simulink model "HDVSim_BEV_Truck"  (R2019b)
settings: Solver=ode3  StartTime=0.0  StopTime=inf  FixedStep=sample_time  MaxStep=0.1  RelTol=1e-3  EnableMultiTasking=on
model workspace (MAT data in the model file):
  Bat : object (value not decoded)
  Electric_Truck = 1
  FuelCell : P_nom (value not decoded)
  Fueltype = 7
  Hybrid_Truck = 1
  IZ12 = 3600
  M_el = 1000
  SOC_T_EM_completely_available = 0.5
  SOC_addition = 0.4
  SOC_el = 0.8
  SOC_target = 0.85
  Sailing_without_drag_torque = 0
  TCO : object (value not decoded)
  TCO_Trailer = 1
  T_distance_LPS_down = 250
  T_distance_LPS_up = 250
  VSim : object (value not decoded)
  Vehicle = 'empty'
  WPT : object (value not decoded)
  acquisitionCosts : acquisitionCosts (value not decoded)
  addition_for_critical_slope = 0.01
  ambient : object (value not decoded)
  auxiliary_consumers : object (value not decoded)
  critical_altitude_difference = 50
  cycle : object (value not decoded)
  dcycle = 22
  distance_1_PPC = 175
  distance_2_PPC = 200
  distance_PPC_altitude_difference = 10000
  driver : object (value not decoded)
  em : object (value not decoded)
  engine : object (value not decoded)
  final_drive : object (value not decoded)
  ifElectric = 1
  ifOptimized = 0
  look_ahead_PPC = 250
  max_distance = 100000
  name = 'HDVSim_BEV_Truck'
  preditiveCruiseControl = 0
  sample_time = 0.1
  tank : object (value not decoded)
  tires : object (value not decoded)
  transmission : object (value not decoded)
  v_PPC_delta = 2.77777777778
  v_max_electrical_drive_only = 13.8888888889
  vehicle : object (value not decoded)
  vehicleProperties : vehicleProperties (value not decoded)
  weights : weights (value not decoded)
  x = 1
values from neighbouring files (symbols this model uses):
  transmission = Transmission_gearing(15.86, 7, 0, 0, final_drive.ratio)    [Parameterizing.m]
symbols that are objects in the model workspace (value not decoded): ambient, auxiliary_consumers, Bat, cycle, driver, em, final_drive, tires, vehicle
undefined symbols (not defined in the file or in its folder): Ion, Lithium, prospective_cruise_control, Vorausschauender_Tempomat
libraries: simulink x21, powerlib x2, electricdrivelib x1
(part 3 of 3)

== system HDVSim_BEV_Truck/Active cruise control_old/Estimate acceleration/Fahrwiderstaende ohne Beschleunigung/drag - Luftwiderstand ==
  v [m/s] : Inport
  A : Constant  Value=vehicle.frontal_area
  Product2 : Product  Inputs=4  RndMeth=Zero
  cW : Constant  Value=vehicle.air_drag_coeff
  gain2 : Gain  Gain=0.5
  rho : Constant  Value=ambient.air_density
  v² : Math  Operator=square  SaturateOnIntegerOverflow=on
  F_Luft [N] : Outport  VectorParamsAs1DForOutWhenUnconnected=off
  wires:
  v²/1 -> Product2/1
  gain2/1 -> F_Luft [N]/1
  v [m/s]/1 -> v²/1
  rho/1 -> Product2/2
  A/1 -> Product2/3
  cW/1 -> Product2/4
  Product2/1 -> gain2/1

== system HDVSim_BEV_Truck/Active cruise control_old/Estimate acceleration/Fahrwiderstaende ohne Beschleunigung/grade resistance - Steigungswiderstand ==
  alpha [rad] : Inport
  Add : Sum
  Constant1 : Constant  Value=vehicle.payload
  Constant2 : Constant  Value=vehicle.mass
  Product7 : Product  RndMeth=Zero
  Trigonometric Function : Trigonometry
  g : Gain  Gain=ambient.gravity
  F_Steig [N] : Outport  VectorParamsAs1DForOutWhenUnconnected=off
  wires:
  alpha [rad]/1 -> Trigonometric Function/1
  Trigonometric Function/1 -> Product7/2
  Product7/1 -> F_Steig [N]/1
  g/1 -> Product7/1
  Constant2/1 -> Add/1
  Constant1/1 -> Add/2
  Add/1 -> g/1

== system HDVSim_BEV_Truck/Active cruise control_old/Estimate acceleration/Fahrwiderstaende ohne Beschleunigung/rolling resistance - Rollwiderstand ==
  alpha [rad] : Inport
  Add1 : Sum
  Constant1 : Constant  Value=vehicle.payload
  Constant5 : Constant  Value=tires.roll_drag_coeff.total
  Constant8 : Constant  Value=vehicle.mass
  Product7 : Product  Inputs=3  RndMeth=Zero
  Trigonometric Function : Trigonometry  Operator=cos
  g : Gain  Gain=ambient.gravity
  F_Roll [N] : Outport  VectorParamsAs1DForOutWhenUnconnected=off
  wires:
  alpha [rad]/1 -> Trigonometric Function/1
  Product7/1 -> F_Roll [N]/1
  Constant5/1 -> Product7/3
  Trigonometric Function/1 -> Product7/1
  g/1 -> Product7/2
  Constant8/1 -> Add1/1
  Constant1/1 -> Add1/2
  Add1/1 -> g/1

== system HDVSim_BEV_Truck/Transmission/Determine when shifting occurs/Gear change recommendation/recommend_down_calcbsfc1 ==
  n_ICE [rpm] : Inport
  shift_parameter.n_2 : Inport  Port=2
  delta_v : Inport  Port=3
  Compare To Constant : simulink/Logic and Bit Operations/Compare To Constant  relop=>=  const=8  OutDataTypeStr=boolean
  Compare To Constant1 : simulink/Logic and Bit Operations/Compare To Constant  relop=>=  const=5  OutDataTypeStr=boolean
  Compare To Zero3 : simulink/Logic and Bit Operations/Compare To Zero  relop=<=  OutDataTypeStr=boolean
  Constant : Constant  Value=em.n_eck
  Constant2 : Constant
  Constant3 : Constant  Value=0
  Display : Display
  Gain : Gain  Gain=3.6
  Gain1 : Gain  Gain=1.05
  Integrator2 : Integrator  ExternalReset=either
  Logical Operator : Logic  Operator=OR  AllPortsSameDT=off  OutDataTypeStr=boolean
  Logical Operator1 : Logic  AllPortsSameDT=off  OutDataTypeStr=boolean
  Relational Operator : RelationalOperator  Operator=<=  OutDataTypeStr=boolean  RndMeth=Nearest
  Scope : Scope  NumInputPorts=3
  Speed jump when downshifiting : Gain  Gain=transmission.ratios(1)/transmission.ratios(2)
  Sum1 : Sum  Inputs=+-|
  Switch1 : Switch  Criteria=u2 > Threshold
  Out1 : Outport  VectorParamsAs1DForOutWhenUnconnected=off
  wires:
  Sum1/1 -> Compare To Zero3/1
  n_ICE [rpm]/1 -> Speed jump when downshifiting/1, Sum1/1
  shift_parameter.n_2/1 -> Sum1/2
  Logical Operator/1 -> Out1/1, Scope/3
  Compare To Zero3/1 -> Logical Operator/1
  delta_v/1 -> Gain/1
  Gain/1 -> Compare To Constant/1
  Integrator2/1 -> Compare To Constant1/1, Display/1
  Switch1/1 -> Integrator2/2, Integrator2/1
  Constant2/1 -> Switch1/1
  Compare To Constant/1 -> Switch1/2
  Constant3/1 -> Switch1/3
  Compare To Constant1/1 -> Scope/2, Logical Operator1/1  "Speed too low"
  Logical Operator1/1 -> Logical Operator/2
  Speed jump when downshifiting/1 -> Relational Operator/1
  Constant/1 -> Gain1/1
  Gain1/1 -> Relational Operator/2
  Relational Operator/1 -> Scope/1, Logical Operator1/2  "Speed jump when downshifiting"

== system HDVSim_BEV_Truck/Transmission/Determine when shifting occurs/Gear change recommendation/recommend_up_calc_bsfc1 ==
  M : Inport
  n_6 : Inport  Port=2
  n_2 : Inport  Port=3
  n : Inport  Port=4
  M_max [Nm] : Inport  Port=5
  v_target [m/s] : Inport  Port=6
  Compare To Zero : simulink/Logic and Bit Operations/Compare To Zero  relop=<=  OutDataTypeStr=boolean
  Compare To Zero1 : simulink/Logic and Bit Operations/Compare To Zero  relop=~=  OutDataTypeStr=boolean
  Logical Operator : Logic  AllPortsSameDT=off  OutDataTypeStr=boolean
  MATLAB Function1 : MATLAB Function  TreatAsAtomicUnit=on
  Sum2 : Sum  Inputs=+-|
  recommend_up : Outport  VectorParamsAs1DForOutWhenUnconnected=off
  wires:
  n_6/1 -> MATLAB Function1/3(n_6)
  n/1 -> MATLAB Function1/1(n)
  n_2/1 -> MATLAB Function1/4(n_2)
  M_max [Nm]/1 -> MATLAB Function1/2(M_max)
  M/1 -> Sum2/1
  Sum2/1 -> Compare To Zero/1
  MATLAB Function1/1(g_2) -> Sum2/2
  v_target [m/s]/1 -> Compare To Zero1/1
  Compare To Zero/1 -> Logical Operator/1
  Compare To Zero1/1 -> Logical Operator/2
  Logical Operator/1 -> recommend_up/1

== stateflow chart HDVSim_BEV_Truck/ECU/Chart ==
  state Hybrid_Truck
    state Accelerating
      state Electric_driving
        during: u_EM = M_required / M_EM_max; u_KB = 0;
      (default) -> (junction 496)
      (junction 496) -> Electric_driving
    state Braking
      state Braking1
        % Conventional braking
        during: u_KB = Driver_B; u_EM = 0;
      state Braking2
        % Regenerative braking, additionally possibly conventional braking
        entry: REKUP = 1;
        exit: REKUP = 0;
        state Braking3
          % Regenerative and conventional braking
          during: u_EM = -1; u_KB = (F_brake_required - F_brake_el_max) / vehicle_F_brake_max;
        state Braking4
          % Regenerative braking
          during: u_EM = -(F_brake_required / F_brake_el_max); u_KB = 0;
        (junction 504) -> Braking3 [order 1] : [F_brake_required > F_brake_el_max]
        Braking4 -> Braking3 : [F_brake_required > F_brake_el_max]
        Braking3 -> Braking4 : [F_brake_required <= F_brake_el_max]
        (default) -> (junction 504)
        (junction 504) -> Braking4 [order 2] : [F_brake_required <= F_brake_el_max]
      (junction 497) -> Braking1 [order 1] : [SOC == 1]
      Braking2 -> Braking1 : [SOC == 1]
      Braking1 -> Braking2 : [SOC < 1]
      (default) -> (junction 497)
      (junction 497) -> Braking2 [order 2]
    state Rolling
      entry: ROLL = 1;
      exit: ROLL = 0;
      state Rolling1
        during: u_EM = 0; u_KB = 0;
      (default) -> Rolling1
    (junction 513) -> Accelerating [order 1] : [Driver_M > 0 && Driver_B == 0]
    (default) -> (junction 513)
    (junction 513) -> Braking [order 2] : [Driver_B > 0 && Driver_M == 0]
    (junction 513) -> Rolling [order 3]
    Braking -> Accelerating [order 1] : [Driver_M > 0 && Driver_B == 0]
    Accelerating -> Braking [order 1] : [Driver_B > 0 && Driver_M == 0]
    Rolling -> Accelerating [order 2] : [Driver_M > 0 && Driver_B == 0]
    Accelerating -> Rolling [order 2] : [Driver_M == 0 && Driver_B == 0]
    Rolling -> Braking [order 1] : [Driver_B > 0 && Driver_M == 0]
    Braking -> Rolling [order 2] : [Driver_M == 0 && Driver_B == 0]
  (junction 222) -> Hybrid_Truck : [Hybrid_Truck == 1]
  (default) -> (junction 222)
  data: u_EM output; Driver_M input; Driver_B input; SOC input; M_EM_max input; M_required input; F_brake_required input; F_brake_el_max input; u_KB output; Hybrid_Truck parameter; ROLL output; REKUP output; vehicle_F_brake_max local =vehicle.F_brake_max

== stateflow chart HDVSim_BEV_Truck/Active cruise control_old/Chart ==
  state Steigung
    entry: Signal_Steigung = 1;
    during: v_vT = 6/3.6;
    exit: Signal_Steigung = 0;
  state Ebene
    during: Signal_Steigung = 0; v_vT = 0;
  state Gefaelle1
    entry: Signal_Gefaelle = 1;
    exit: Signal_Gefaelle = 0;
  Ebene -> Steigung [order 2] : [Steigung_500 > Kritische_Steigung &&...
      | Steigung_700 > Kritische_Steigung &&...
      | Vorausschauender_Tempomat == 1]
  Steigung -> Ebene : [Steigung_50 <= Kritische_Steigung &&...
      | Steigung_0 <= Kritische_Steigung &&...
      | Zurueckgelegte_Strecke > 500]
  (default) -> Ebene
  Ebene -> Gefaelle1 [order 1] : [(Beschleunigung_0 +...
      | Beschleunigung_50 +...
      | Beschleunigung_100 +...
      | Beschleunigung_150 +...
      | Beschleunigung_200)/5 >= -0.17 &&...
      | (Beschleunigung_250 +...
      | Beschleunigung_300 +...
      | Beschleunigung_350 +...
      | Beschleunigung_400 +...
      | Beschleunigung_450)/5 >= 0.17 &&...
      | Fahrer_M > 0 &&...
      | Vorausschauender_Tempomat == 1]
  Gefaelle1 -> Ebene : [Zurueckgelegte_Strecke_2 > 450 ||...
      | Fahrer_B > 0]
  data: Kritische_Steigung input; Beschleunigung_0 input; Beschleunigung_50 input; Beschleunigung_100 input; Beschleunigung_150 input; Beschleunigung_200 input; Beschleunigung_250 input; Beschleunigung_300 input; Beschleunigung_350 input; Beschleunigung_400 input; Beschleunigung_450 input; Steigung_0 input; Steigung_50 input; Steigung_100 input; Steigung_250 input; Steigung_350 input; Steigung_500 input; Steigung_700 input; Fahrer_M input; Fahrer_B input; Zurueckgelegte_Strecke input; Zurueckgelegte_Strecke_2 input; v_vT output double; Signal_Steigung output double; Signal_Gefaelle output double; Vorausschauender_Tempomat parameter

== stateflow chart HDVSim_BEV_Truck/Transmission/Shifting rules ==
  state gear_state [parallel]
    settings: executionOrder=1
    state gear016
      entry: gear=16;
    state gear015
      entry: gear=15;
    state gear014
      entry: gear=14;
    state gear013
      entry: gear=13;
    state gear012
      entry: gear=12;
    state gear011
      entry: gear=11;
    state gear010
      entry: gear=10;
    state gear09
      entry: gear=9;
    state gear08
      entry: gear=8;
    state gear07
      entry: gear=7;
    state gear06
      entry: gear=6;
    state gear05
      entry: gear=5;
    state gear04
      entry: gear=4;
    state gear03
      entry: gear=3;
    state gear02
      entry: gear=2;
    state gear01
      entry: gear=1;
    gear015 -> gear016 [order 3] : TWO_UP
    gear016 -> gear014 [order 2] : TWO_DOWN
    gear014 -> gear016 [order 3] : TWO_UP
    (junction 349) -> gear016 [order 16] : [init_gear==16]
    gear016 -> gear015 [order 1] : DOWN
    gear015 -> gear016 [order 1] : UP
    gear015 -> gear013 [order 4] : TWO_DOWN
    (junction 349) -> gear015 [order 15] : [init_gear==15]
    gear013 -> gear015 [order 3] : TWO_UP
    gear015 -> gear014 [order 2] : DOWN
    gear014 -> gear015 [order 1] : UP
    gear014 -> gear012 [order 4] : TWO_DOWN
    gear012 -> gear014 [order 4] : TWO_UP
    (junction 349) -> gear014 [order 14] : [init_gear==14]
    gear014 -> gear013 [order 2] : DOWN
    gear013 -> gear014 [order 1] : UP
    gear011 -> gear013 [order 4] : TWO_UP
    gear013 -> gear011 [order 4] : TWO_DOWN
    (junction 349) -> gear013 [order 13] : [init_gear==13]
    gear013 -> gear012 [order 2] : DOWN
    gear012 -> gear013 [order 3] : UP
    (junction 349) -> gear012 [order 12] : [init_gear==12]
    gear010 -> gear012 [order 4] : TWO_UP
    gear012 -> gear010 [order 2] : TWO_DOWN
    gear012 -> gear011 [order 1] : DOWN
    gear011 -> gear012 [order 1] : UP
    gear011 -> gear09 [order 3] : TWO_DOWN
    gear09 -> gear011 [order 4] : TWO_UP
    (junction 349) -> gear011 [order 11] : [init_gear==11]
    gear011 -> gear010 [order 2] : DOWN
    gear010 -> gear011 [order 1] : UP
    gear08 -> gear010 [order 4] : TWO_UP
    gear010 -> gear08 [order 3] : TWO_DOWN
    (junction 349) -> gear010 [order 10] : [init_gear==10]
    gear010 -> gear09 [order 2] : DOWN
    gear09 -> gear010 [order 1] : UP
    gear07 -> gear09 [order 4] : TWO_UP
    gear09 -> gear07 [order 3] : TWO_DOWN
    (junction 349) -> gear09 [order 9] : [init_gear==9]
    gear09 -> gear08 [order 2] : DOWN
    gear08 -> gear09 [order 2] : UP
    gear06 -> gear08 [order 4] : TWO_UP
    gear08 -> gear06 [order 3] : TWO_DOWN
    (junction 349) -> gear08 [order 8] : [init_gear==8]
    gear08 -> gear07 [order 1] : DOWN
    gear07 -> gear08 [order 3] : UP
    gear07 -> gear05 [order 2] : TWO_DOWN
    gear05 -> gear07 [order 4] : TWO_UP
    (junction 349) -> gear07 [order 7] : [init_gear==7]
    gear07 -> gear06 [order 1] : DOWN
    gear06 -> gear07 [order 3] : UP
    (junction 349) -> gear06 [order 6] : [init_gear==6]
    gear06 -> gear04 [order 2] : TWO_DOWN
    (junction 349) -> gear01 [order 1] : [init_gear==1]
    (junction 349) -> gear05 [order 5] : [init_gear==5]
    gear04 -> gear06 [order 3] : TWO_UP
    (junction 349) -> gear02 [order 2] : [init_gear==2]
    (junction 349) -> gear04 [order 4] : [init_gear==4]
    (junction 349) -> gear03 [order 3] : [init_gear==3]
    gear06 -> gear05 [order 1] : DOWN
    gear05 -> gear06 [order 1] : UP
    gear05 -> gear03 [order 3] : TWO_DOWN
    gear03 -> gear05 [order 3] : TWO_UP
    gear05 -> gear04 [order 2] : DOWN
    gear04 -> gear05 [order 1] : UP
    gear04 -> gear02 [order 4] : TWO_DOWN
    gear02 -> gear04 [order 3] : TWO_UP
    gear04 -> gear03 [order 2] : DOWN
    gear03 -> gear04 [order 1] : UP
    gear01 -> gear03 [order 2] : TWO_UP
    gear03 -> gear01 [order 4] : TWO_DOWN
    gear03 -> gear02 [order 2] : DOWN
    gear02 -> gear03 [order 1] : UP
    gear02 -> gear01 [order 4] : TWO_DOWN
    gear02 -> gear01 [order 2] : DOWN
    gear01 -> gear02 [order 1] : UP
  state selection_state [parallel]
    settings: executionOrder=2
    state upshift2
      entry: TWO_UP;
      exit: wait_state.WAIT;
    state upshift1
      entry: UP;
      exit: wait_state.WAIT;
    note: 2: UP due to recommendation
        | 3: UP due to speed max
    state steady_state
    note: 1: DOWN due to recommendation
        | 4: DOWN due to torque maximum
        | 5: DOWN due to speed min
    state downshift1
      entry: DOWN;
      exit: wait_state.WAIT;
    state downshift2
      entry: TWO_DOWN;
      exit: wait_state.WAIT;
    upshift2 -> steady_state
    (junction 405) -> upshift2 [order 1] : [recommend_down_2higher==0]
    (junction 405) -> upshift1 [order 2] : [recommend_down_2higher==1]
    (junction 404) -> (junction 405) [order 1] : [check_torque_reserve_2higher==1]
    (junction 404) -> upshift1 [order 2] : [check_torque_reserve_2higher==0]
    (junction 403) -> (junction 404) [order 1] : [check_n_min_2higher==1 && check_M_max_2higher==1]
    (junction 403) -> upshift1 [order 2] : [check_n_min_2higher==0 || check_M_max_2higher==0]
    (junction 380) -> (junction 403) [order 1] : [recommend_up_1higher==1 && gear<=z-2]
    (junction 380) -> upshift1 [order 2] : [recommend_up_1higher==0 || gear>z-2]
    steady_state -> upshift1 [order 3] : [check_n_max_now==0 && gear<=z-1]
    upshift1 -> steady_state
    steady_state -> (junction 380) [order 2] : [(recommend_up_now==1 && check_n_max_now==1) && check_n_min_1higher==1 && check_M_max_1higher==1 && gear<=z-1 && waiting3s==0]
    (default) -> steady_state
    downshift1 -> steady_state
    downshift2 -> steady_state
    steady_state -> (junction 367) [order 1] : [(recommend_down_now==1 && check_M_max_now==1 && check_n_min_now==1) && check_n_max_1lower==1 && gear>=2 && waiting3s==0]
    steady_state -> downshift1 [order 4] : [(check_M_max_now==0 && check_n_min_now==1) && check_n_max_1lower==1 &&gear>=2 && check_n_min_now==1 && waiting3s==0]
    steady_state -> downshift1 [order 5] : [(check_n_min_now==0)&& gear>3]
    (junction 367) -> downshift1 [order 1] : [recommend_down_1lower==0 || gear<3]
    (junction 367) -> (junction 394) [order 2] : [recommend_down_1lower==1 && gear>=3]
    (junction 394) -> downshift1 [order 2] : [check_n_max_2lower==0]
    (junction 394) -> (junction 397) [order 1] : [check_n_max_2lower==1]
    (junction 397) -> downshift1 [order 2] : [recommend_up_2lower==1]
    (junction 397) -> downshift2 [order 1] : [recommend_up_2lower==0]
  state wait_state [parallel]
    settings: executionOrder=3
    state shifting_ready
      entry: waiting3s=0;
    state wait3s
      entry: waiting3s=1;
    shifting_ready -> wait3s : WAIT
    (default) -> shifting_ready
    wait3s -> shifting_ready : after(3,sec)
  (default) -> (junction 349)
  data: gear output uint8; waiting3s local double; init_gear input double; z input double; recommend_down_2higher input boolean; recommend_down_1higher input boolean; recommend_down_now input boolean; recommend_down_1lower input boolean; recommend_down_2llower input boolean; recommend_up_2higher input boolean; recommend_up_1higher input boolean; recommend_up_now input boolean; recommend_up_1lower input boolean; recommend_up_2lower input boolean; check_n_min_2higher input boolean; check_n_min_1higher input boolean; check_n_min_now input boolean; check_n_min_1lower input boolean; check_n_min_2lower input boolean; check_n_max_2higher input boolean; check_n_max_1higher input boolean; check_n_max_now input boolean; check_n_max_1lower input boolean; check_n_max_2lower input boolean; check_M_max_2higher input boolean; check_M_max_1higher input boolean; check_M_max_now input boolean; check_M_max_1lower input boolean; check_M_max_2lower input boolean; check_torque_reserve_2higher input boolean; check_torque_reserve_2lower input boolean
  events: WAIT local EITHER_EDGE_EVENT; DOWN local EITHER_EDGE_EVENT; TWO_DOWN local EITHER_EDGE_EVENT; TWO_UP local EITHER_EDGE_EVENT; UP local EITHER_EDGE_EVENT

== stateflow chart HDVSim_BEV_Truck/Active cruise control1/Chart ==
  state Incline
    entry: Signal_incline = 1;
    exit: Signal_incline = 0;
  state Even
  state Decline
    entry: Signal_decline = 1;
    exit: Signal_decline = 0;
  Even -> Incline [order 2] : [look_ahead_PPC > critical_incline &&...
      | look_ahead_PPC+distance_PPC > critical_incline &&...
      | prospective_cruise_control == 1]
  Incline -> Even : [incline_0 < critical_incline &&...
      | incline_100 < critical_incline &&...
      | incline_200 < critical_incline &&...
      | incline_300 < critical_incline &&...
      | incline_400 < critical_incline &&...
      | incline_500 < critical_incline &&...
      | Distance_covered > look_ahead_PPC+distance_PPC]
  (default) -> Even
  Even -> Decline [order 1] : [(Acceleration_0 +...
      | Acceleration_50 +...
      | Acceleration_100 +...
      | Acceleration_150 +...
      | Acceleration_200)/5 >= -(v_max_cycle/distance_2_PPC*v_PPC_delta) &&...
      | (Acceleration_250 +...
      | Acceleration_300 +...
      | Acceleration_350 +...
      | Acceleration_400 +...
      | Acceleration_450)/5 >= (v_max_cycle/distance_2_PPC*v_PPC_delta) &&...
      | Driver_M > 0 &&...
      | prospective_cruise_control == 1 &&...
      | v_current >= 60/3.6]
  Decline -> Even : [Distance_covered_2 > 450 ||...
      | Driver_B > 0]
  data: critical_incline input; Acceleration_0 input; Acceleration_50 input; Acceleration_100 input; Acceleration_150 input; Acceleration_200 input; Acceleration_250 input; Acceleration_300 input; Acceleration_350 input; Acceleration_400 input; Acceleration_450 input; incline_0 input; incline_100 input; incline_200 input; incline_300 input; incline_400 input; incline_500 input; Driver_M input; Driver_B input; Distance_covered input; Distance_covered_2 input; Signal_incline output double; Signal_decline output double; prospective_cruise_control constant double =preditiveCruiseControl; v_PPC_delta constant double; v_max_cycle constant double; distance_2_PPC constant double; distance_PPC constant double; look_ahead_PPC constant double; v_current input

== matlab function HDVSim_BEV_Truck/Transmission/Determine when shifting occurs/Gear change recommendation/recommend_up_calc_bsfc1/MATLAB Function1 ==
  data: n input; g_2 output; M_max input; n_6 input; n_2 input
function g_2 = fcn(n,M_max,n_6,n_2)
%#codegen

g_2 = M_max / (n_6 - n_2) * (n - n_2);

== stateflow chart HDVSim_BEV_Truck/Active cruise control2/Chart1 ==
  state Incline
    entry: Signal_incline = 1;
    exit: Signal_incline = 0;
  state Even
  state Decline
    entry: Signal_decline = 1;
    exit: Signal_decline = 0;
  Even -> Incline [order 2] : [look_ahead_PPC > critical_incline &&...
      | look_ahead_PPC+distance_PPC > critical_incline &&...
      | prospective_cruise_control == 1]
  Incline -> Even : [incline_0 < critical_incline &&...
      | incline_100 < critical_incline &&...
      | incline_200 < critical_incline &&...
      | incline_300 < critical_incline &&...
      | incline_400 < critical_incline &&...
      | incline_500 < critical_incline &&...
      | Distance_covered > look_ahead_PPC+distance_PPC]
  (default) -> Even
  Even -> Decline [order 1] : [(Acceleration_0 +...
      | Acceleration_50 +...
      | Acceleration_100 +...
      | Acceleration_150 +...
      | Acceleration_200)/5 >= -(v_max_cycle/distance_2_PPC*v_PPC_delta) &&...
      | (Acceleration_250 +...
      | Acceleration_300 +...
      | Acceleration_350 +...
      | Acceleration_400 +...
      | Acceleration_450)/5 >= (v_max_cycle/distance_2_PPC*v_PPC_delta) &&...
      | Driver_M > 0 &&...
      | prospective_cruise_control == 1 &&...
      | v_current >= 60/3.6]
  Decline -> Even : [Distance_covered_2 > 450 ||...
      | Driver_B > 0]
  data: critical_incline input; Acceleration_0 input; Acceleration_50 input; Acceleration_100 input; Acceleration_150 input; Acceleration_200 input; Acceleration_250 input; Acceleration_300 input; Acceleration_350 input; Acceleration_400 input; Acceleration_450 input; incline_0 input; incline_100 input; incline_200 input; incline_300 input; incline_400 input; incline_500 input; incline_distance_look_ahead_min input; incline_distance_look_ahead_max input; Driver_M input; Driver_B input; Distance_covered input; Distance_covered_2 input; Signal_incline output double; Signal_decline output double; prospective_cruise_control constant double =preditiveCruiseControl; look_ahead constant double; v_PPC_delta constant double; v_max_cycle constant double; distance constant double; distance_2_PPC constant double; distance_PPC constant double; look_ahead_PPC constant double; v_current input
